simulink model "PruebaMotores"  (R2022a)
settings: Solver=FixedStepAuto  StartTime=0.0  StopTime=30  RelTol=1e-3  EnableMultiTasking=on
libraries: slpidlib x1
settings Model: SimulationMode=external  ExtModeTrigDuration=2  Creator=Laura Sierra Ruiz  LastModifiedBy=Nuc1
settings OptimizationCC: EnhancedBackFolding=on  PassReuseOutputArgsAs=Individual arguments  ZeroExternalMemoryAtStartup=off  ZeroInternalMemoryAtStartup=off  MaxStackSize=64  OptimizeBlockOrder=speed  DifferentSizesBufferReuse=on  OptimizationCustomize=off  EfficientTunableParamExpr=on
settings DebuggingCC: ParameterTunabilityLossMsg=error  UnconnectedInputMsg=warning  UnconnectedOutputMsg=warning  UnconnectedLineMsg=warning
settings HardwareCC: ProdBitPerInt=16  ProdBitPerPointer=16  ProdBitPerSizeT=16  ProdBitPerPtrDiffT=16  ProdLargestAtomicFloat=None  ProdWordSize=8  ProdHWDeviceType=Atmel->AVR
settings SFSimCC: MATLABDynamicMemAlloc=off
settings RTWCC: SystemTargetFile=ert.tlc  HardwareBoard=Arduino Mega 2560  TemplateMakefile=ert_default_tmf  Toolchain=Arduino AVR  BuildConfiguration=Faster Runs  DLArmComputeVersion=19.05
settings CodeAppCC: ForceParamTrailComments=on  IgnoreCustomStorageClasses=off  OperatorAnnotations=on  SimulinkDataObjDesc=on  SFDataObjDesc=on  InsertBlockDesc=on
settings ERTTargetCC: SupportContinuousTime=on  SupportVariableSizeSignals=on  ExtMode=on  ExtModeTransport=3  ExtModeStaticAlloc=on  ExtModeStaticAllocSize=2048  ExtModeMexFile=ext_xcp  ExtModeMexArgs=0 3 921600  ExtModeIntrfLevel=Level2 - Open

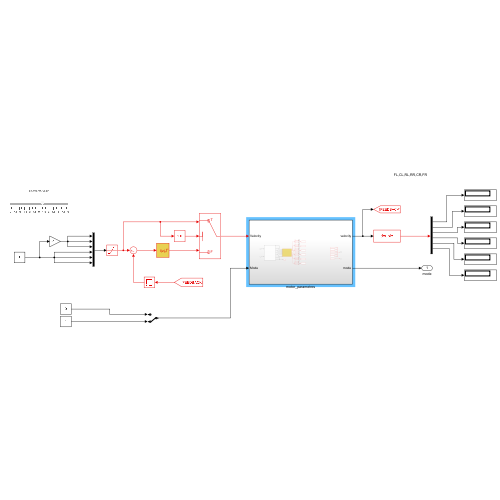
[thumbnail: Simulink's stored preview of the top-level diagram]
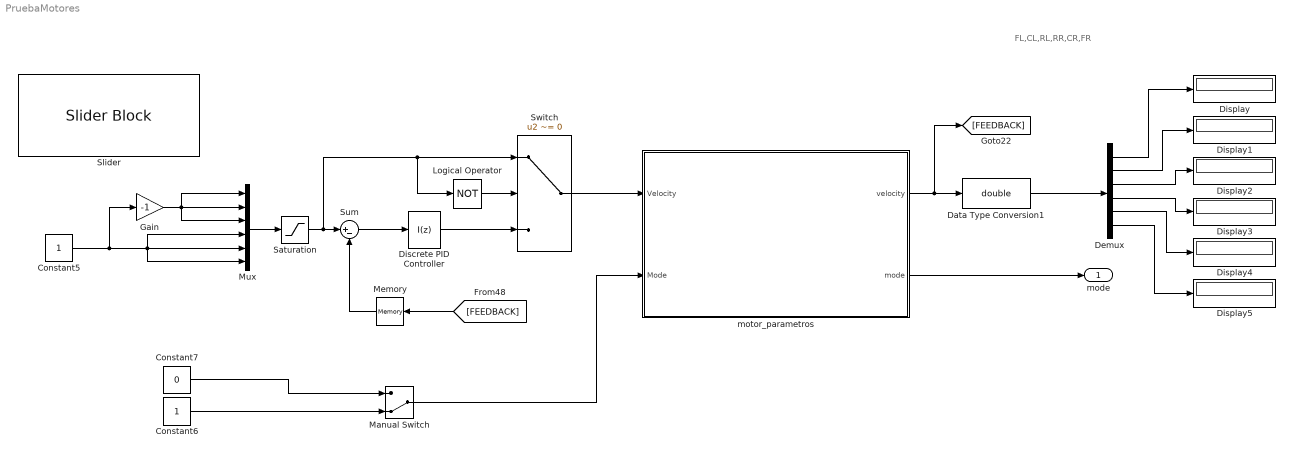
== system PruebaMotores ==
  note: FL,CL,RL,RR,CR,FR
  Constant5 : Constant
  Constant6 : Constant
  Constant7 : Constant  Value=0
  Data Type Conversion1 : DataTypeConversion  OutDataTypeStr=double  SaturateOnIntegerOverflow=off  RndMeth=Floor
  Demux : Demux  Outputs=6
  Discrete PID Controller : slpidlib/PID Controller  Controller=I  Form=Parallel  TimeDomain=Discrete-time  UseExternalTs=off  SampleTime=-1  IntegratorMethod=Forward Euler  FilterMethod=Forward Euler  ControllerParametersSource=internal  P=0.7  I=10  UseKiTs=off  D=0  N=100  UseFilter=on  TunerSelectOption=Transfer Function Based (PID Tuner App)  InitialConditionSource=internal  InitialConditionForIntegrator=0  InitialConditionForFilter=0  DifferentiatorICPrevScaledInput=0  ExternalReset=none  TrackingMode=off  Kt=1  LimitOutput=on  SatLimitsSource=internal  UpperSaturationLimit=10  LowerSaturationLimit=-10  LinearizeAsGain=on  AntiWindupMode=clamping  Kb=1  POutMin=[]  POutMax=[]  IOutMin=[]  IOutMax=[]  DOutMin=[]  DOutMax=[]  NOutMin=[]  NOutMax=[]  SumOutMin=[]  SumOutMax=[]  SaturationOutMin=[]  SaturationOutMax=[]  PParamMin=[]  PParamMax=[]  IParamMin=[]  IParamMax=[]  DParamMin=[]  DParamMax=[]  NParamMin=[]  NParamMax=[]  KbParamMin=[]  KbParamMax=[]  KtParamMin=[]  KtParamMax=[]  KbOutMin=[]  KbOutMax=[]  KtOutMin=[]  KtOutMax=[]  IntegratorOutMin=[]  IntegratorOutMax=[]  FilterOutMin=[]  FilterOutMax=[]  SumI1OutMin=[]  SumI1OutMax=[]  SumI2OutMin=[]  SumI2OutMax=[]  SumI3OutMin=[]  SumI3OutMax=[]  SumI4OutMin=[]  SumI4OutMax=[]  SumDOutMin=[]  SumDOutMax=[]  DifferentiatorOutMin=[]  DifferentiatorOutMax=[]  FilterDiffOutCoefMin=[]  FilterDiffOutCoefMax=[]  ReciprocalOutMin=[]  ReciprocalOutMax=[]  SumDenOutMin=[]  SumDenOutMax=[]  SumNumOutMin=[]  SumNumOutMax=[]  DivideOutMin=[]  DivideOutMax=[]  UdiffTsProdOutMin=[]  UdiffTsProdOutMax=[]  NTsProdOutMin=[]  NTsProdOutMax=[]  UintegralTsProdOutMin=[]  UintegralTsProdOutMax=[]  UngainTsProdOutMin=[]  UngainTsProdOutMax=[]  IntegratorContinuousStateAttributes=''  IntegratorStateMustResolveToSignalObject=off  IntegratorRTWStateStorageClass=Auto  FilterContinuousStateAttributes=''  FilterStateMustResolveToSignalObject=off  FilterRTWStateStorageClass=Auto  ParallelPVariant=Disabled  IdealPVariant=Disabled  IVariant=InternalParameters  DVariant=Disabled  IntegratorVariant=Discrete  SatVariant=Enabled  AWVariant=DiscClampingParallel  PCopyVariant=Disabled  TRVariant=Disabled  FdbkBlocksVariant=Forward  IdealPFdbkVariant=Disabled  SatFdbkVariant=Disabled  DerivativeFilterVariant=Disabled  NVariant=Disabled  NCopyVariant=Disabled_SignalSpec  FilterICVariant=Disabled  IntegratorICVariant=InternalICs  ExternalResetVariant=Disabled  TRSumVariant=Passthrough  SumFdbkVariant=Disabled  SumVariant=Passthrough_I  TsampFilterVariant=InternalTs  TsampNgainVariant=Passthrough  TsampIntegralVariant=Passthrough  ExternalSaturationOutDataTypeStr=Inherit: Same as second input  aMode=0
  Display{,1..5} (6 alike) : Display
  Gain : Gain  Gain=-1
  Logical Operator : Logic  Operator=NOT  AllPortsSameDT=off  OutDataTypeStr=boolean
  Manual Switch : ManualSwitch  CurrentSetting=0
  Memory : Memory
  Mux : Mux  Inputs=6
  Saturation : Saturate  UpperLimit=10  LowerLimit=-10
  Slider : SliderBlock  ScaleMin=-9  ScaleMax=9
  Sum : Sum  Inputs=|+-
  Switch : Switch  Criteria=u2 ~= 0  SaturateOnIntegerOverflow=off  InputSameDT=off
  motor_parametros : Subsystem
  mode : Outport
  wires:
  Switch/1 -> motor_parametros/1(Velocity)
  Saturation/1 -> Logical Operator/1, Switch/1, Sum/1
  motor_parametros/1(velocity) -> [FEEDBACK], Data Type Conversion1/1
  Logical Operator/1 -> Switch/2
  [FEEDBACK] -> Memory/1
  Data Type Conversion1/1 -> Demux/1
  motor_parametros/2(mode) -> mode/1
  Discrete PID Controller/1 -> Switch/3
  Sum/1 -> Discrete PID Controller/1
  Memory/1 -> Sum/2
  Mux/1 -> Saturation/1
  Gain/1 -> Mux/1, Mux/2, Mux/3
  Constant5/1 -> Gain/1, Mux/6, Mux/4, Mux/5
  Demux/1 -> Display/1
  Demux/2 -> Display1/1
  Demux/3 -> Display2/1
  Demux/4 -> Display3/1
  Demux/5 -> Display4/1
  Demux/6 -> Display5/1
  Constant6/1 -> Manual Switch/2
  Constant7/1 -> Manual Switch/1
  Manual Switch/1 -> motor_parametros/2(Mode)

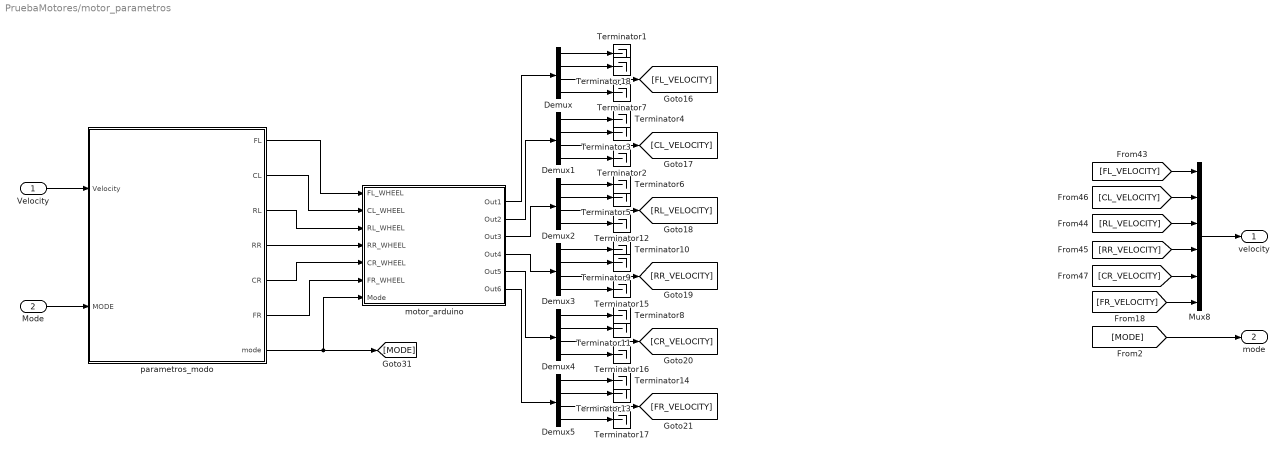
== system PruebaMotores/motor_parametros ==
  Velocity : Inport
  Mode : Inport  Port=2
  Demux{,1..5} (6 alike) : Demux
  Mux8 : Mux  Inputs=6
  Terminator{1..18} (18 alike) : Terminator
  motor_arduino : Subsystem
      mask Display: image('motor.jpg'); % Use "Edit Image" on toolstrip to change.
  parametros_modo : Subsystem
  velocity : Outport
  mode : Outport  Port=2
  wires:
  [CL_VELOCITY] -> Mux8/2
  [FR_VELOCITY] -> Mux8/6
  Demux4/1 -> Terminator8/1
  parametros_modo/6(FR) -> motor_arduino/6(FR_WHEEL)
  [RL_VELOCITY] -> Mux8/3
  Demux/1 -> Terminator1/1
  parametros_modo/2(CL) -> motor_arduino/2(CL_WHEEL)
  parametros_modo/5(CR) -> motor_arduino/5(CR_WHEEL)
  Demux1/3 -> [CL_VELOCITY]
  motor_arduino/5(Out5) -> Demux4/1
  parametros_modo/1(FL) -> motor_arduino/1(FL_WHEEL)
  motor_arduino/3(Out3) -> Demux2/1
  [RR_VELOCITY] -> Mux8/4
  parametros_modo/4(RR) -> motor_arduino/4(RR_WHEEL)
  Demux2/3 -> [RL_VELOCITY]
  Demux1/2 -> Terminator3/1
  motor_arduino/1(Out1) -> Demux/1
  parametros_modo/3(RL) -> motor_arduino/3(RL_WHEEL)
  Demux3/2 -> Terminator9/1
  Demux/2 -> Terminator18/1
  [CR_VELOCITY] -> Mux8/5
  [FL_VELOCITY] -> Mux8/1
  Demux2/2 -> Terminator5/1
  Demux/3 -> [FL_VELOCITY]
  Demux3/3 -> [RR_VELOCITY]
  Demux1/1 -> Terminator4/1
  Demux3/1 -> Terminator10/1
  motor_arduino/2(Out2) -> Demux1/1
  Demux4/3 -> [CR_VELOCITY]
  Demux5/2 -> Terminator13/1
  motor_arduino/4(Out4) -> Demux3/1
  Demux2/1 -> Terminator6/1
  motor_arduino/6(Out6) -> Demux5/1
  Demux5/3 -> [FR_VELOCITY]
  Demux5/1 -> Terminator14/1
  Demux4/2 -> Terminator11/1
  Mux8/1 -> velocity/1
  Velocity/1 -> parametros_modo/1(Velocity)
  Mode/1 -> parametros_modo/2(MODE)
  parametros_modo/7(mode) -> [MODE], motor_arduino/7(Mode)
  [MODE] -> mode/1
  Demux1/4 -> Terminator2/1
  Demux/4 -> Terminator7/1
  Demux2/4 -> Terminator12/1
  Demux3/4 -> Terminator15/1
  Demux4/4 -> Terminator16/1
  Demux5/4 -> Terminator17/1

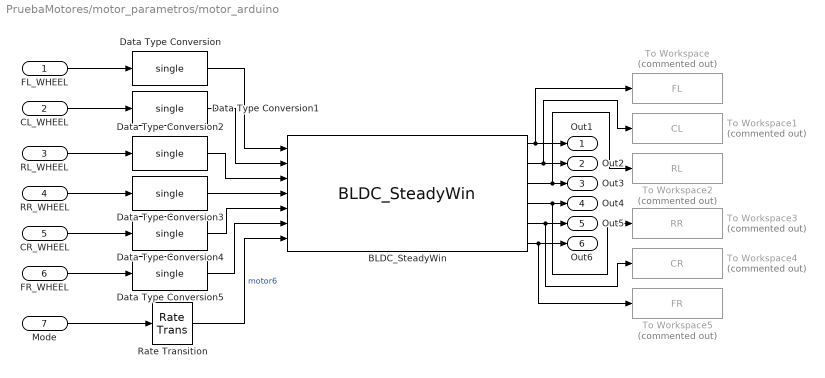
== system PruebaMotores/motor_parametros/motor_arduino ==
  FL_WHEEL : Inport
  CL_WHEEL : Inport  Port=2
  RL_WHEEL : Inport  Port=3
  RR_WHEEL : Inport  Port=4
  CR_WHEEL : Inport  Port=5
  FR_WHEEL : Inport  Port=6
  Mode : Inport  Port=7
  BLDC_SteadyWin : S-Function  InitFcn=try, set_param(gcb,'FunctionName','BLDC_SteadyWin'), end  FunctionName=BLDC_SteadyWin  SFunctionModules=BLDC_SteadyWin_wrapper  SFunctionDeploymentMode=off  EnableBusSupport=off  mask(S-Function Builder){}
      mask help: Simulink:masks:SFunctionBuilder_MD
      mask init:
      | val = [[.9  0.75 0.75 1 1 .9 .9 1]',[1 1 0.75 0.75 .9 .9 1 .9]'];try , sys = get_param(gcb,'SfunBuilderFcnName');if isempty(sys), sys = get_param(gcb,'FunctionName'); end,catch, sys = get_param(gcb,'FunctionName'); end
      settings: CopyFcn=set_param(gcbh,'LinkStatus','none')  PreSaveFcn=try, set_param(gcb,'FunctionName','BLDC_SteadyWin'), end  OpenFcn=sfunctionwizard(gcbh)
      mask Display:
      | plot(val(:,1),val(:,2))
      | disp(sys)
      | port_label('input',1,'In1')
      | port_label('input',2,'In2')
      | port_label('input',3,'In3')
      | port_label('input',4,'In4')
      | port_label('input',5,'In5')
      | port_label('input',6,'In6')
      | port_label('input',7,'Mode')
      | port_label('output',1,'Out1')
      | port_label('output',2,'Out2')
      | port_label('output',3,'Out3')
      | port_label('output',4,'Out4')
      | port_label('output',5,'Out5')
      | port_label('output',6,'Out6')
  Data Type Conversion{,1..5} (6 alike) : DataTypeConversion  OutDataTypeStr=single  SaturateOnIntegerOverflow=off  RndMeth=Floor
  Rate Transition : RateTransition
  To Workspace : ToWorkspace  Commented=on  VariableName=FL  SaveFormat=Structure With Time  SampleTime=-1
  To Workspace1 : ToWorkspace  Commented=on  VariableName=CL  SaveFormat=Structure With Time  SampleTime=-1
  To Workspace2 : ToWorkspace  Commented=on  VariableName=RL  SaveFormat=Structure With Time  SampleTime=-1
  To Workspace3 : ToWorkspace  Commented=on  VariableName=RR  SaveFormat=Structure With Time  SampleTime=-1
  To Workspace4 : ToWorkspace  Commented=on  VariableName=CR  SaveFormat=Structure With Time  SampleTime=-1
  To Workspace5 : ToWorkspace  Commented=on  VariableName=FR  SaveFormat=Structure With Time  SampleTime=-1
  Out1 : Outport
  Out2 : Outport  Port=2
  Out3 : Outport  Port=3
  Out4 : Outport  Port=4
  Out5 : Outport  Port=5
  Out6 : Outport  Port=6
  wires:
  FL_WHEEL/1 -> Data Type Conversion/1
  BLDC_SteadyWin/1 -> To Workspace/1, Out1/1
  BLDC_SteadyWin/2 -> To Workspace1/1, Out2/1
  BLDC_SteadyWin/3 -> To Workspace2/1, Out3/1
  BLDC_SteadyWin/4 -> To Workspace3/1, Out4/1
  BLDC_SteadyWin/5 -> To Workspace4/1, Out5/1
  BLDC_SteadyWin/6 -> To Workspace5/1, Out6/1
  CL_WHEEL/1 -> Data Type Conversion1/1
  Data Type Conversion1/1 -> BLDC_SteadyWin/2
  Data Type Conversion/1 -> BLDC_SteadyWin/1
  Mode/1 -> Rate Transition/1
  Data Type Conversion3/1 -> BLDC_SteadyWin/4
  Data Type Conversion2/1 -> BLDC_SteadyWin/3
  RL_WHEEL/1 -> Data Type Conversion2/1
  RR_WHEEL/1 -> Data Type Conversion3/1
  Data Type Conversion5/1 -> BLDC_SteadyWin/6
  Data Type Conversion4/1 -> BLDC_SteadyWin/5
  CR_WHEEL/1 -> Data Type Conversion4/1
  FR_WHEEL/1 -> Data Type Conversion5/1
  Rate Transition/1 -> BLDC_SteadyWin/7  "motor6"

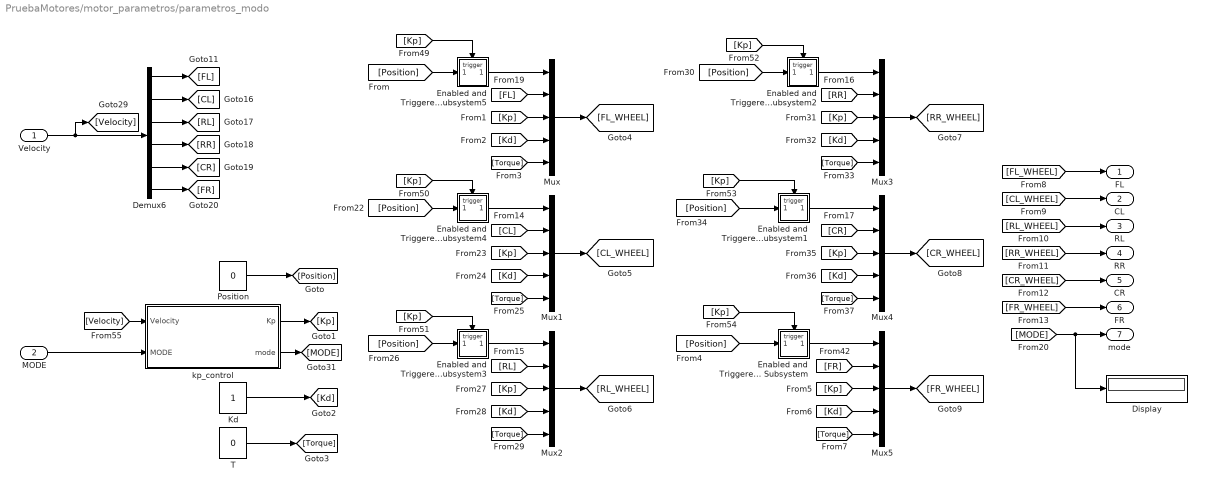
== system PruebaMotores/motor_parametros/parametros_modo ==
  Velocity : Inport
  MODE : Inport  Port=2
  Demux6 : Demux  Outputs=6
  Display : Display
  Enabled and Triggered Subsystem : Subsystem  TreatAsAtomicUnit=on
  Enabled and Triggered Subsystem1 : Subsystem  TreatAsAtomicUnit=on
  Enabled and Triggered Subsystem2 : Subsystem  TreatAsAtomicUnit=on
  Enabled and Triggered Subsystem3 : Subsystem  TreatAsAtomicUnit=on
  Enabled and Triggered Subsystem4 : Subsystem  TreatAsAtomicUnit=on
  Enabled and Triggered Subsystem5 : Subsystem  TreatAsAtomicUnit=on
  Kd : Constant  SampleTime=-1
  Mux{,1..5} (6 alike) : Mux  Inputs=5
  Position : Constant  Value=0  SampleTime=-1
  T : Constant  Value=0  SampleTime=-1
  kp_control : Subsystem
  FL : Outport
  CL : Outport  Port=2
  RL : Outport  Port=3
  RR : Outport  Port=4
  CR : Outport  Port=5
  FR : Outport  Port=6
  mode : Outport  Port=7
  wires:
  [Kp] -> Mux/3
  [RR] -> Mux3/2
  [Kp] -> Mux3/3
  [Torque] -> Mux3/5
  [Torque] -> Mux4/5
  [RL] -> Mux2/2
  Enabled and Triggered Subsystem3/1(Out1) -> Mux2/1
  [Kd] -> Mux2/4
  Mux1/1 -> [CL_WHEEL]
  [Kp] -> Mux4/3
  [Torque] -> Mux1/5
  [Kd] -> Mux1/4
  Mux5/1 -> [FR_WHEEL]
  [Kp] -> Mux1/3
  Mux2/1 -> [RL_WHEEL]
  [CR] -> Mux4/2
  [Torque] -> Mux2/5
  [FL] -> Mux/2
  [Kd] -> Mux/4
  Mux4/1 -> [CR_WHEEL]
  [Position] -> Enabled and Triggered Subsystem1/1(In1)
  [Kd] -> Mux4/4
  [Kp] -> Mux2/3
  [Torque] -> Mux/5
  Enabled and Triggered Subsystem4/1(Out1) -> Mux1/1
  Enabled and Triggered Subsystem/1(Out1) -> Mux5/1
  Mux3/1 -> [RR_WHEEL]
  Enabled and Triggered Subsystem5/1(Out1) -> Mux/1
  [Kd] -> Mux3/4
  [CL] -> Mux1/2
  [Kd] -> Mux5/4
  [Position] -> Enabled and Triggered Subsystem5/1(In1)
  [Position] -> Enabled and Triggered Subsystem/1(In1)
  [Kp] -> Enabled and Triggered Subsystem1/Trigger
  [FR] -> Mux5/2
  [Kp] -> Enabled and Triggered Subsystem4/Trigger
  Enabled and Triggered Subsystem1/1(Out1) -> Mux4/1
  [Position] -> Enabled and Triggered Subsystem2/1(In1)
  [Torque] -> Mux5/5
  [Kp] -> Enabled and Triggered Subsystem3/Trigger
  [Position] -> Enabled and Triggered Subsystem4/1(In1)
  [Kp] -> Mux5/3
  [Position] -> Enabled and Triggered Subsystem3/1(In1)
  Mux/1 -> [FL_WHEEL]
  [Kp] -> Enabled and Triggered Subsystem5/Trigger
  [Kp] -> Enabled and Triggered Subsystem/Trigger
  Enabled and Triggered Subsystem2/1(Out1) -> Mux3/1
  [Kp] -> Enabled and Triggered Subsystem2/Trigger
  Demux6/6 -> [FR]
  Demux6/1 -> [FL]
  kp_control/2(mode) -> [MODE]
  MODE/1 -> kp_control/2(MODE)
  Kd/1 -> [Kd]
  T/1 -> [Torque]
  Position/1 -> [Position]
  kp_control/1(Kp) -> [Kp]
  [Velocity] -> kp_control/1(Velocity)
  Velocity/1 -> Demux6/1, [Velocity]
  [FL_WHEEL] -> FL/1
  [CL_WHEEL] -> CL/1
  [RL_WHEEL] -> RL/1
  [RR_WHEEL] -> RR/1
  [CR_WHEEL] -> CR/1
  [FR_WHEEL] -> FR/1
  [MODE] -> Display/1, mode/1
  Demux6/2 -> [CL]
  Demux6/3 -> [RL]
  Demux6/4 -> [RR]
  Demux6/5 -> [CR]

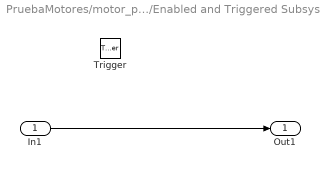
== system PruebaMotores/motor_parametros/parametros_modo/Enabled and Triggered Subsystem ==
  In1 : Inport
  Trigger : TriggerPort  VariantControl=Variant
  Out1 : Outport
  wires:
  In1/1 -> Out1/1

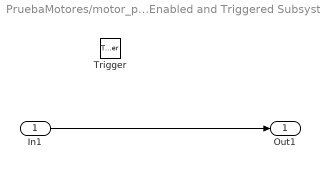
== system PruebaMotores/motor_parametros/parametros_modo/Enabled and Triggered Subsystem1 ==
  In1 : Inport
  Trigger : TriggerPort  VariantControl=Variant
  Out1 : Outport
  wires:
  In1/1 -> Out1/1

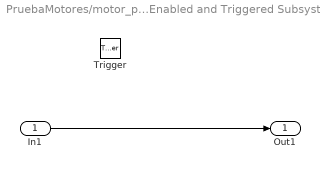
== system PruebaMotores/motor_parametros/parametros_modo/Enabled and Triggered Subsystem2 ==
  In1 : Inport
  Trigger : TriggerPort  VariantControl=Variant
  Out1 : Outport
  wires:
  In1/1 -> Out1/1

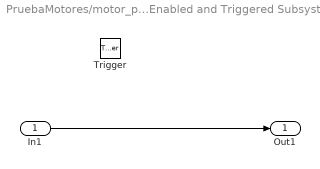
== system PruebaMotores/motor_parametros/parametros_modo/Enabled and Triggered Subsystem3 ==
  In1 : Inport
  Trigger : TriggerPort  VariantControl=Variant
  Out1 : Outport
  wires:
  In1/1 -> Out1/1

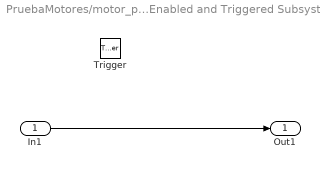
== system PruebaMotores/motor_parametros/parametros_modo/Enabled and Triggered Subsystem4 ==
  In1 : Inport
  Trigger : TriggerPort  VariantControl=Variant
  Out1 : Outport
  wires:
  In1/1 -> Out1/1

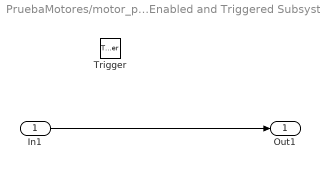
== system PruebaMotores/motor_parametros/parametros_modo/Enabled and Triggered Subsystem5 ==
  In1 : Inport
  Trigger : TriggerPort  VariantControl=Variant
  Out1 : Outport
  wires:
  In1/1 -> Out1/1

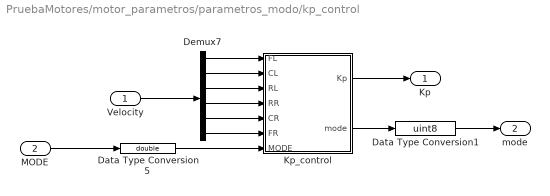
== system PruebaMotores/motor_parametros/parametros_modo/kp_control ==
  Velocity : Inport
  MODE : Inport  Port=2
  Data Type Conversion1 : DataTypeConversion  OutDataTypeStr=uint8  SaturateOnIntegerOverflow=off  RndMeth=Floor
  Data Type Conversion5 : DataTypeConversion  OutDataTypeStr=double  SaturateOnIntegerOverflow=off  RndMeth=Floor
  Demux7 : Demux  Outputs=6
  Kp_control : MATLAB Function  TreatAsAtomicUnit=on
  Kp : Outport
  mode : Outport  Port=2
  wires:
  Demux7/5 -> Kp_control/5(CR)
  Demux7/6 -> Kp_control/6(FR)
  Demux7/1 -> Kp_control/1(FL)
  Demux7/2 -> Kp_control/2(CL)
  Kp_control/1(Kp) -> Kp/1
  Demux7/3 -> Kp_control/3(RL)
  Demux7/4 -> Kp_control/4(RR)
  Velocity/1 -> Demux7/1
  Kp_control/2(mode) -> Data Type Conversion1/1
  Data Type Conversion1/1 -> mode/1
  MODE/1 -> Data Type Conversion5/1
  Data Type Conversion5/1 -> Kp_control/7(MODE)

== matlab function PruebaMotores/motor_parametros/parametros_modo/kp_control/Kp_control ==
  data: FL input; Kp output; CL input; RL input; RR input; CR input; FR input; MODE input size=1; mode output
function [Kp, mode] = fcn(FL,CL,RL,RR,CR,FR,MODE)

    if(FL==0) && (CL==0) && (RL==0) && (RR==0) && (CR==0) && (FR==0) && (MODE==1)
        Kp = 25;
        mode = 2;
    else
        Kp = 0;
        mode = MODE;
    end
